simulink model "admittance_control"  (R2021b)
settings: Solver=FixedStepAuto  StartTime=0.0  StopTime=5  FixedStep=Ts  RelTol=1e-3
undefined symbols (not defined in the file): dqi, K, KD, KDt, KP, KPt, Mt, myRobot, qf, qi, qr, xr
libraries: vrlib x1
settings Model: Creator=simon  LastModifiedBy=luigi
settings SolverCC: ZeroCrossControl=DisableAll  AlgebraicLoopSolver=TrustRegion
settings DebuggingCC: SFMachineParentedDataDiag=warning

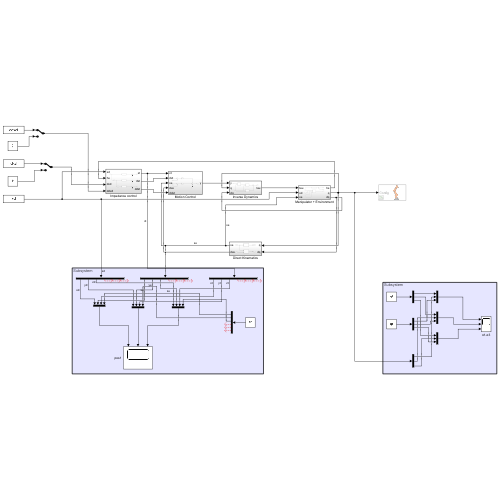
[thumbnail: Simulink's stored preview of the top-level diagram]
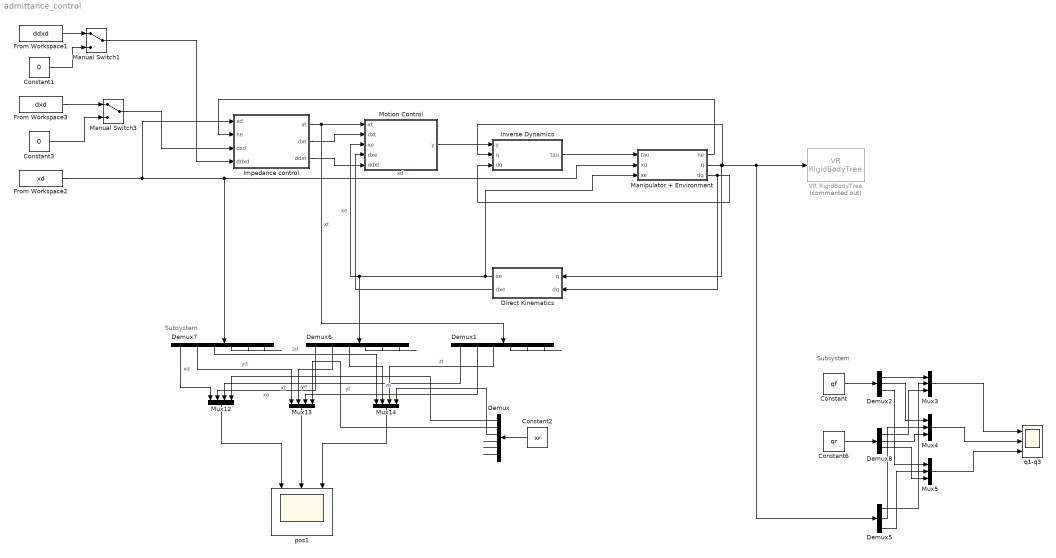
== system admittance_control ==
  note: Subsystem
  note: Subsystem
  Constant : Constant  Value=qf
  Constant1 : Constant  Value=0
  Constant2 : Constant  Value=xr
  Constant3 : Constant  Value=0
  Constant6 : Constant  Value=qr
  Demux{,1,6..7} (4 alike) : Demux  Outputs=6
  Demux2 : Demux  Outputs=3
  Demux5 : Demux  Outputs=myRobot.N
  Demux8 : Demux  Outputs=3
  Direct Kinematics : Subsystem
  From Workspace1 : FromWorkspace  VariableName=ddxd
  From Workspace2 : FromWorkspace  VariableName=xd
  From Workspace3 : FromWorkspace  VariableName=dxd
  Impedance control : Subsystem
  Inverse Dynamics : Subsystem
  Manipulator + Environment : Subsystem
  Manual Switch1 : ManualSwitch
  Manual Switch3 : ManualSwitch
  Motion Control : Subsystem
  Mux12 : Mux
  Mux13 : Mux
  Mux14 : Mux
  Mux3 : Mux  Inputs=3
  Mux4 : Mux  Inputs=3
  Mux5 : Mux  Inputs=3
  VR RigidBodyTree : vrlib/VR RigidBodyTree  Commented=on  RBT=rbt  useRBT=on  Ts=-1  ForceViewerOpen=on
      settings: SourceProductBaseCode=SL
  pos1 : Scope  NumInputPorts=3
  q1-q3 : Scope  NumInputPorts=3
  wires:
  Inverse Dynamics/1(tau) -> Manipulator + Environment/1(tau)
  Manipulator + Environment/3(dq) -> Inverse Dynamics/3(dq), Direct Kinematics/2(dq)
  Manipulator + Environment/1(he) -> Impedance control/2(he)
  From Workspace3/1 -> Manual Switch3/1
  Constant3/1 -> Manual Switch3/2
  Direct Kinematics/1(xe) -> Demux6/1, Motion Control/3(xe), Manipulator + Environment/3(xe)  "xe"
  From Workspace2/1 -> Manipulator + Environment/2(xd), Demux7/1, Impedance control/1(xd)  "xd"
  Impedance control/1(xt) -> Demux1/1, Motion Control/1(xt)  "xt"
  Motion Control/1(y) -> Inverse Dynamics/1(y)
  Direct Kinematics/2(dxe) -> Motion Control/4(dxe)
  From Workspace1/1 -> Manual Switch1/1
  Constant1/1 -> Manual Switch1/2
  Manual Switch3/1 -> Impedance control/3(dxd)
  Manual Switch1/1 -> Impedance control/4(ddxd)
  Impedance control/2(dxt) -> Motion Control/2(dxt)
  Impedance control/3(ddxt) -> Motion Control/5(ddxt)
  Demux6/4 -> ?
  Demux6/5 -> ?
  Demux6/6 -> ?
  Demux7/6 -> ?
  Demux1/6 -> ?
  Demux1/4 -> ?
  Demux/4 -> ?
  Demux/5 -> ?
  Demux/3 -> Mux14/4
  Demux7/5 -> ?
  Demux/2 -> Mux13/4
  Demux7/3 -> Mux14/1  "zd"
  Demux/6 -> ?
  Constant2/1 -> Demux/1
  Mux12/1 -> pos1/1
  Demux6/3 -> Mux14/2  "ze"
  Mux14/1 -> pos1/3
  Mux13/1 -> pos1/2
  Demux/1 -> Mux12/4
  Demux1/5 -> ?
  Demux1/1 -> Mux12/3  "xt"
  Demux7/1 -> Mux12/1  "xd"
  Demux1/2 -> Mux13/3  "yt"
  Demux7/4 -> ?
  Demux1/3 -> Mux14/3  "zt"
  Demux6/2 -> Mux13/2  "ye"
  Demux6/1 -> Mux12/2  "xe"
  Demux7/2 -> Mux13/1  "yd"
  Manipulator + Environment/2(q) -> Demux5/1, VR RigidBodyTree/1, Inverse Dynamics/2(q), Direct Kinematics/1(q)
  Constant/1 -> Demux2/1
  Demux5/1 -> Mux3/2
  Demux2/1 -> Mux3/1
  Demux5/2 -> Mux4/2
  Mux3/1 -> q1-q3/1
  Demux2/2 -> Mux4/1
  Demux8/1 -> Mux3/3
  Demux5/3 -> Mux5/2
  Demux8/3 -> Mux5/3
  Mux5/1 -> q1-q3/3
  Demux2/3 -> Mux5/1
  Demux8/2 -> Mux4/3
  Mux4/1 -> q1-q3/2
  Constant6/1 -> Demux8/1

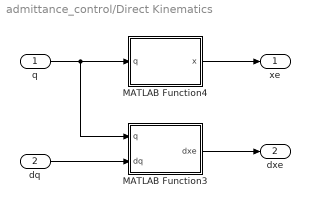
== system admittance_control/Direct Kinematics ==
  q : Inport
  dq : Inport  Port=2
  MATLAB Function3 : MATLAB Function  TreatAsAtomicUnit=on
  MATLAB Function4 : MATLAB Function  TreatAsAtomicUnit=on
  xe : Outport
  dxe : Outport  Port=2
  wires:
  MATLAB Function3/1(dxe) -> dxe/1
  dq/1 -> MATLAB Function3/2(dq)
  q/1 -> MATLAB Function3/1(q), MATLAB Function4/1(q)
  MATLAB Function4/1(x) -> xe/1

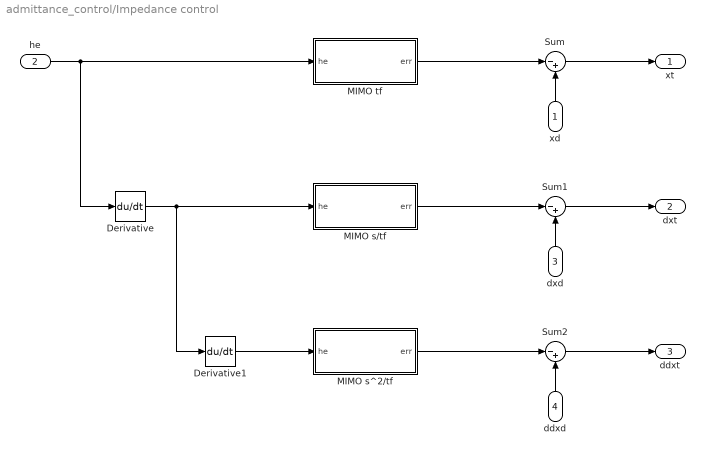
== system admittance_control/Impedance control ==
  xd : Inport
  he : Inport  Port=2
  dxd : Inport  Port=3
  ddxd : Inport  Port=4
  Derivative : Derivative
  Derivative1 : Derivative
  MIMO s/tf : Subsystem
  MIMO s^2/tf : Subsystem
  MIMO tf : Subsystem
  Sum : Sum  Inputs=|-+
  Sum1 : Sum  Inputs=|-+
  Sum2 : Sum  Inputs=|-+
  xt : Outport
  dxt : Outport  Port=2
  ddxt : Outport  Port=3
  wires:
  xd/1 -> Sum/2
  Sum/1 -> xt/1
  he/1 -> Derivative/1, MIMO tf/1(he)
  MIMO tf/1(err) -> Sum/1
  dxd/1 -> Sum1/2
  Sum1/1 -> dxt/1
  MIMO s/tf/1(err) -> Sum1/1
  ddxd/1 -> Sum2/2
  Sum2/1 -> ddxt/1
  MIMO s^2/tf/1(err) -> Sum2/1
  Derivative/1 -> MIMO s/tf/1(he), Derivative1/1
  Derivative1/1 -> MIMO s^2/tf/1(he)

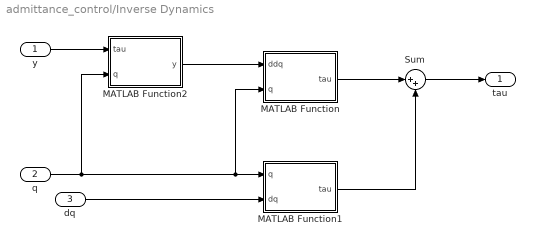
== system admittance_control/Inverse Dynamics ==
  y : Inport
  q : Inport  Port=2
  dq : Inport  Port=3
  MATLAB Function : MATLAB Function  TreatAsAtomicUnit=on
  MATLAB Function1 : MATLAB Function  TreatAsAtomicUnit=on
  MATLAB Function2 : MATLAB Function  TreatAsAtomicUnit=on
  Sum : Sum  Inputs=|++
  tau : Outport
  wires:
  MATLAB Function1/1(tau) -> Sum/2
  MATLAB Function/1(tau) -> Sum/1
  Sum/1 -> tau/1
  dq/1 -> MATLAB Function1/2(dq)
  q/1 -> MATLAB Function/2(q), MATLAB Function1/1(q), MATLAB Function2/2(q)
  y/1 -> MATLAB Function2/1(tau)
  MATLAB Function2/1(y) -> MATLAB Function/1(ddq)

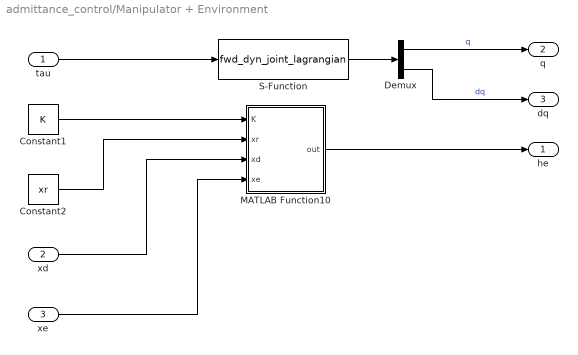
== system admittance_control/Manipulator + Environment ==
  tau : Inport
  xd : Inport  Port=2
  xe : Inport  Port=3
  Constant1 : Constant  Value=K
  Constant2 : Constant  Value=xr
  Demux : Demux  Outputs=2
  MATLAB Function10 : MATLAB Function  TreatAsAtomicUnit=on
  S-Function : S-Function  FunctionName=fwd_dyn_joint_lagrangian  Parameters=myRobot,qi,dqi  SFunctionDeploymentMode=off  EnableBusSupport=off
  he : Outport
  q : Outport  Port=2
  dq : Outport  Port=3
  wires:
  tau/1 -> S-Function/1
  Constant1/1 -> MATLAB Function10/1(K)
  Constant2/1 -> MATLAB Function10/2(xr)
  xd/1 -> MATLAB Function10/3(xd)
  xe/1 -> MATLAB Function10/4(xe)
  S-Function/1 -> Demux/1
  Demux/1 -> q/1  "q"
  Demux/2 -> dq/1  "dq"
  MATLAB Function10/1(out) -> he/1

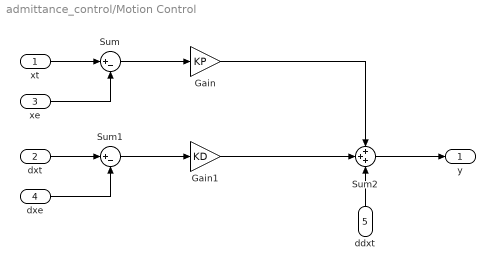
== system admittance_control/Motion Control ==
  xt : Inport
  dxt : Inport  Port=2
  xe : Inport  Port=3
  dxe : Inport  Port=4
  ddxt : Inport  Port=5
  Gain : Gain  Gain=KP
  Gain1 : Gain  Gain=KD
  Sum : Sum  Inputs=|+-
  Sum1 : Sum  Inputs=|+-
  Sum2 : Sum  Inputs=+++
  y : Outport
  wires:
  xt/1 -> Sum/1
  xe/1 -> Sum/2
  Sum/1 -> Gain/1
  dxt/1 -> Sum1/1
  dxe/1 -> Sum1/2
  Sum1/1 -> Gain1/1
  Gain/1 -> Sum2/1
  Gain1/1 -> Sum2/2
  Sum2/1 -> y/1
  ddxt/1 -> Sum2/3

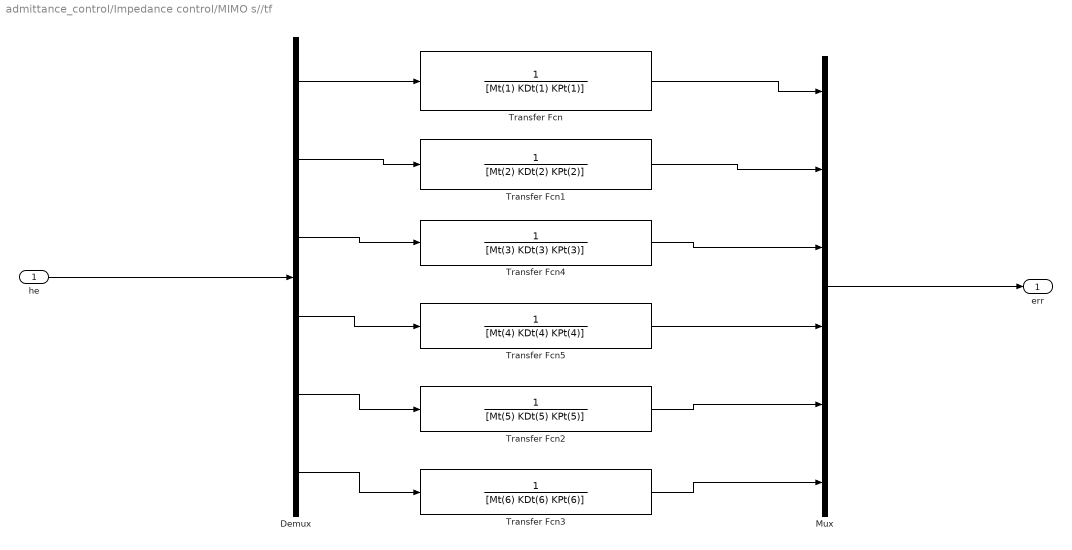
== system admittance_control/Impedance control/MIMO s//tf ==
  he : Inport
  Demux : Demux  Outputs=6
  Mux : Mux  Inputs=6
  Transfer Fcn : TransferFcn  Denominator=[Mt(1) KDt(1) KPt(1)]
  Transfer Fcn1 : TransferFcn  Denominator=[Mt(2) KDt(2) KPt(2)]
  Transfer Fcn2 : TransferFcn  Denominator=[Mt(5) KDt(5) KPt(5)]
  Transfer Fcn3 : TransferFcn  Denominator=[Mt(6) KDt(6) KPt(6)]
  Transfer Fcn4 : TransferFcn  Denominator=[Mt(3) KDt(3) KPt(3)]
  Transfer Fcn5 : TransferFcn  Denominator=[Mt(4) KDt(4) KPt(4)]
  err : Outport
  wires:
  Demux/4 -> Transfer Fcn5/1
  Transfer Fcn5/1 -> Mux/4
  Transfer Fcn3/1 -> Mux/6
  Transfer Fcn1/1 -> Mux/2
  Transfer Fcn2/1 -> Mux/5
  Mux/1 -> err/1
  Demux/3 -> Transfer Fcn4/1
  Demux/6 -> Transfer Fcn3/1
  Demux/2 -> Transfer Fcn1/1
  he/1 -> Demux/1
  Transfer Fcn/1 -> Mux/1
  Demux/1 -> Transfer Fcn/1
  Transfer Fcn4/1 -> Mux/3
  Demux/5 -> Transfer Fcn2/1

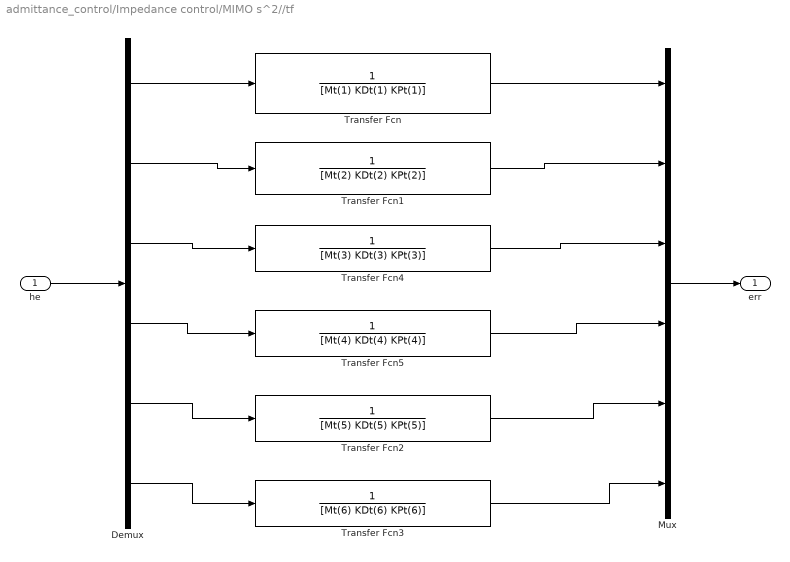
== system admittance_control/Impedance control/MIMO s^2//tf ==
  he : Inport
  Demux : Demux  Outputs=6
  Mux : Mux  Inputs=6
  Transfer Fcn : TransferFcn  Denominator=[Mt(1) KDt(1) KPt(1)]
  Transfer Fcn1 : TransferFcn  Denominator=[Mt(2) KDt(2) KPt(2)]
  Transfer Fcn2 : TransferFcn  Denominator=[Mt(5) KDt(5) KPt(5)]
  Transfer Fcn3 : TransferFcn  Denominator=[Mt(6) KDt(6) KPt(6)]
  Transfer Fcn4 : TransferFcn  Denominator=[Mt(3) KDt(3) KPt(3)]
  Transfer Fcn5 : TransferFcn  Denominator=[Mt(4) KDt(4) KPt(4)]
  err : Outport
  wires:
  Demux/4 -> Transfer Fcn5/1
  Transfer Fcn5/1 -> Mux/4
  Transfer Fcn3/1 -> Mux/6
  Transfer Fcn1/1 -> Mux/2
  Transfer Fcn2/1 -> Mux/5
  Mux/1 -> err/1
  Demux/3 -> Transfer Fcn4/1
  Demux/6 -> Transfer Fcn3/1
  Demux/2 -> Transfer Fcn1/1
  he/1 -> Demux/1
  Transfer Fcn/1 -> Mux/1
  Demux/1 -> Transfer Fcn/1
  Transfer Fcn4/1 -> Mux/3
  Demux/5 -> Transfer Fcn2/1

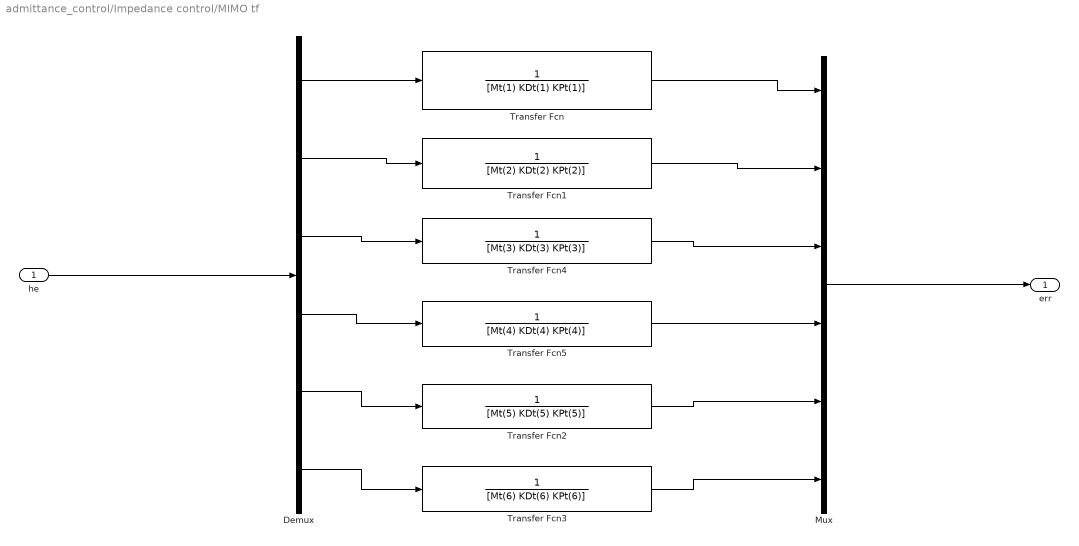
== system admittance_control/Impedance control/MIMO tf ==
  he : Inport
  Demux : Demux  Outputs=6
  Mux : Mux  Inputs=6
  Transfer Fcn : TransferFcn  Denominator=[Mt(1) KDt(1) KPt(1)]
  Transfer Fcn1 : TransferFcn  Denominator=[Mt(2) KDt(2) KPt(2)]
  Transfer Fcn2 : TransferFcn  Denominator=[Mt(5) KDt(5) KPt(5)]
  Transfer Fcn3 : TransferFcn  Denominator=[Mt(6) KDt(6) KPt(6)]
  Transfer Fcn4 : TransferFcn  Denominator=[Mt(3) KDt(3) KPt(3)]
  Transfer Fcn5 : TransferFcn  Denominator=[Mt(4) KDt(4) KPt(4)]
  err : Outport
  wires:
  Demux/4 -> Transfer Fcn5/1
  Transfer Fcn5/1 -> Mux/4
  Transfer Fcn3/1 -> Mux/6
  Transfer Fcn1/1 -> Mux/2
  Transfer Fcn2/1 -> Mux/5
  Mux/1 -> err/1
  Demux/3 -> Transfer Fcn4/1
  Demux/6 -> Transfer Fcn3/1
  Demux/2 -> Transfer Fcn1/1
  he/1 -> Demux/1
  Transfer Fcn/1 -> Mux/1
  Demux/1 -> Transfer Fcn/1
  Transfer Fcn4/1 -> Mux/3
  Demux/5 -> Transfer Fcn2/1

== matlab function admittance_control/Direct Kinematics/MATLAB Function3 ==
  data: q input; dxe output; dq input
function dxe = Ja(q, dq)

dxe = getJa(q)*dq;

== matlab function admittance_control/Inverse Dynamics/MATLAB Function2 ==
  data: tau input; q input; y output
function y = invJa(tau, q)

y = getInvJa(q)*tau;

== matlab function admittance_control/Direct Kinematics/MATLAB Function4 ==
  data: q input; x output
function x = k(q)

x = getK(q);

== matlab function admittance_control/Inverse Dynamics/MATLAB Function ==
  data: ddq input size=3; q input size=3; tau output
function tau = B(ddq, q)

tau = getB(q)*ddq;

== matlab function admittance_control/Inverse Dynamics/MATLAB Function1 ==
  data: q input size=3; tau output; dq input size=3
function tau = n(q, dq)

tau = getN(q, dq);

== matlab function admittance_control/Manipulator + Environment/MATLAB Function10 ==
  data: K input; out output size=6; xr input; xd input; xe input size=6
function out = hde(K, xr, xd, xe)
%consider the interaction only in z direction
% if the end effector touch the environment 
he = zeros(6,1);

if xe(3) < xr(3)
    %The interaction force between the end-effector and the environment is
    dxrd = xd-xr;
    dxed = xd-xe;
    dxre = dxrd-dxed;
    he = K*dxre;
end

out = he;
